simulink model "ss1_inter"  (R2019a)
settings: Solver=ode14x  StartTime=beginTime  StopTime=0.456  FixedStep=1e-4  RelTol=1e-3  EnableMultiTasking=on
model workspace (MAT data in the model file):
  Ankle_L_D = 1.86999822456
  Ankle_L_S = 0.0237763920936
  Ankle_R_D = 0.0588397140494
  Ankle_R_S = 0.739584271752
  F_C = 0.06105
  F_H = 0.07
  F_I = 0.00125071180063
  F_L = 0.185
  F_M = 1.13129
  F_W = 0.1
  GRF_HD = 42097.5090581
  GRF_HS = 111995.804745
  GRF_VD = 23523.4518935
  GRF_VS = 88551.3661398
  HAT_I = 3.41998320224
  HAT_L = 0.51264
  HAT_M = 52.89756
  HAT_a = 0.2
  HAT_b = 0.11
  Hip_L_D = 0.00120944164738
  Hip_L_S = 1.91959156409
  Hip_R_D = 0.00174333284727
  Hip_R_S = 0.483982271561
  Knee_L_D = 0.900041230997
  Knee_L_S = 0.0187606009115
  Knee_R_D = 0.0722123401531
  Knee_R_S = 0.0187606009115
  M : struct (value not decoded)
  S_I = 0.0556212184297
  S_L = 0.41
  S_M = 3.62793
  S_R1 = 0.035
  S_R2 = 0.0716197243914
  T_I = 0.63371745
  T_L = 0.6
  T_M = 7.802
  T_R1 = 0.0716197243914
  T_R2 = 0.105042262441
  beginTime = 0.4399
  bodymass = 78.02
  lagStanceAnkle = [0 0 0 0 0 0]
  lagSwingAnkle = [0 0 0 0 0 0]
  lagSwingHip = [0 0 0 0 0 0]
  lagSwingKnee = [0 0 0 0 0 0]
  p_stance_ankle_i = 17.5320951874
  p_stance_hip_i = 9.45550537668
  p_stance_knee_i = -16.7757020207
  p_swing_ankle_i = -28.2787898978
  p_swing_hip_i = -5.22071177476
  p_swing_knee_i = -39.2892116907
  polyfit_stance_ankle = [7.25005766341 -2.94260084728 3.61751641686 -0.1600680665]
  polyfit_swing_ankle = [-11368.0037517 20285.4827832 -14825.218273 5697.61347658 -1221.0674564 140.988649334 -7.60353693637 0.110238664523]
  polyfit_swing_hip = [-6497.04836191 6353.1189755 -1512.41069047 -218.046365216 114.745718447 -9.14187395017 -0.14056630138]
  polyfit_swing_knee = [20801.7792641 -51031.8985583 53804.8965773 -29864.6420618 9069.83319333 -1458.09150169 107.955966741 -2.65469998779 0.0787369748099]
  w_stance_ankle_i = 0.530344461508
  w_stance_hip_i = -152.886101178
  w_stance_knee_i = 28.9894830902
  w_swing_ankle_i = -177.193414919
  w_swing_hip_i = 0.0149454586906
  w_swing_knee_i = 289.013531197
  x_planar_p_i = -0.0011974861006
  x_planar_v_i = 0.0137263009297
  y_planar_p_i = 0.0112183968788
  y_planar_v_i = -0.080280250047
  z_planar_p_i = 11.2224967124
  z_planar_v_i = -77.4143532804
symbols that are objects in the model workspace (value not decoded): M
undefined symbols (not defined in the file or in its folder): X, Y, Z
libraries: nesl_utility x54, sm_lib x46, fl_lib x24, fl_ps_legacy_lib x14
(part 5 of 7)

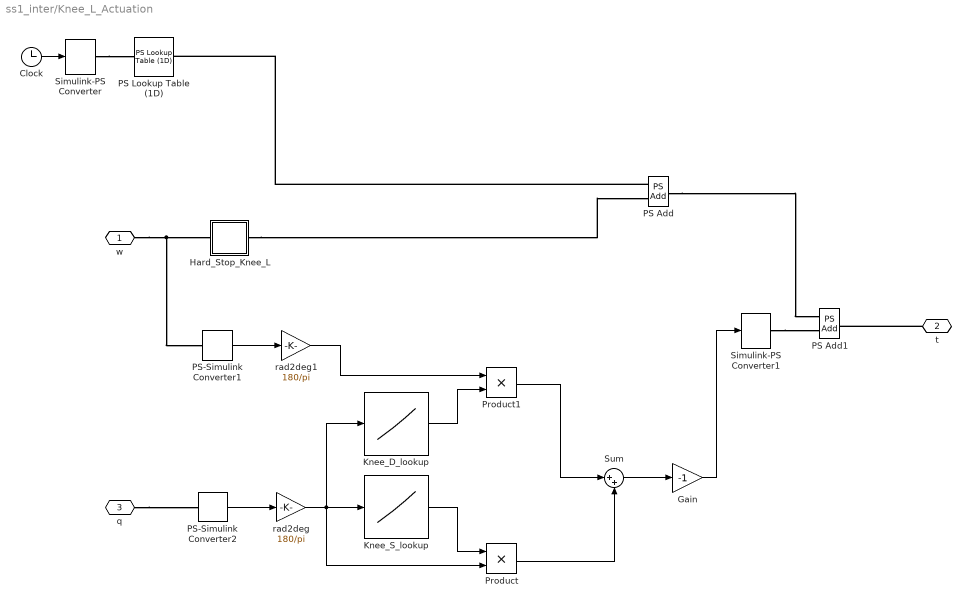
== system ss1_inter/Knee_L_Actuation ==
  Clock : Clock
  Gain : Gain  Gain=-1
  Hard_Stop_Knee_L : Subsystem  mask{upper_bound=(-p_stance_knee_i*pi)/180, lower_bound=((-140-p_stance_knee_i)*pi)/180, contact_stiffness=1e8, contact_damping=5000, initial_angular_position=0}
      mask prompts: upper_bound "Upper Bound"; lower_bound "Lower Bound"; contact_stiffness "Contact Stiffness"; contact_damping "Contact Damping"; initial_angular_position "Initial Angular Position"
  Knee_D_lookup : Lookup_n-D  NumberOfTableDimensions=1  BreakpointsForDimension1=[-140:.01:0]  Table=[exp(linspace(log(1000),log(.01),1000)), zeros(1,12000),exp(linspace(log(.01),log(1000),1001))]  RndMeth=Simplest  InputSameDT=on
  Knee_S_lookup : Lookup_n-D  NumberOfTableDimensions=1  BreakpointsForDimension1=[-140:.01:0]  Table=[exp(linspace(log(10000),log(.01),1000)), zeros(1,12000),exp(linspace(log(.01),log(10000),1001))]  RndMeth=Simplest  InputSameDT=on
  PS Add : fl_ps_legacy_lib/Legacy Physical Signals/Functions/PS Add
      settings: SourceProductName=Simscape  SourceProductBaseCode=SS
  PS Add1 : fl_ps_legacy_lib/Legacy Physical Signals/Functions/PS Add
      settings: SourceProductName=Simscape  SourceProductBaseCode=SS
  PS Lookup Table (1D) : fl_ps_legacy_lib/Legacy Physical Signals/Lookup Tables/PS Lookup Table (1D)  x=linspace(0,.3917,47)'  f=(-M.stance_knee_av/1000)*bodymass  interp_method=2  extrap_method=1
      settings: SourceProductName=Simscape  SourceProductBaseCode=SS
  PS-Simulink Converter1 : nesl_utility/PS-Simulink Converter  PhysicalDomain=network_engine_domain  SubClassName=ps_output  LeftPortType=input  RightPortType=output  PseudoPeriodic=off  Frequencies=[]  Unit=1  AffineConversion=off
  PS-Simulink Converter2 : nesl_utility/PS-Simulink Converter  PhysicalDomain=network_engine_domain  SubClassName=ps_output  LeftPortType=input  RightPortType=output  PseudoPeriodic=off  Frequencies=[]  Unit=1  AffineConversion=off
  Product : Product  RndMeth=Zero
  Product1 : Product  RndMeth=Zero
  Simulink-PS Converter : nesl_utility/Simulink-PS Converter  PhysicalDomain=network_engine_domain  SubClassName=ps_input  LeftPortType=input  RightPortType=output  PseudoPeriodic=off  Frequencies=[]  NoiseDistribution=none  NoiseParameters=[]  Unit=1  AffineConversion=off  FilteringAndDerivatives=zero  SimscapeFilterOrder=1  InputFilterTimeConstant=.001  UdotUserProvided=[]
  Simulink-PS Converter1 : nesl_utility/Simulink-PS Converter  PhysicalDomain=network_engine_domain  SubClassName=ps_input  LeftPortType=input  RightPortType=output  PseudoPeriodic=off  Frequencies=[]  NoiseDistribution=none  NoiseParameters=[]  Unit=1  AffineConversion=off  FilteringAndDerivatives=zero  SimscapeFilterOrder=1  InputFilterTimeConstant=.001  UdotUserProvided=[]
  Sum : Sum  Inputs=|++
  rad2deg : Gain  Gain=180/pi
  "rad2deg1 " : Gain  Gain=180/pi
  w : PMIOPort  Side=Right
  t : PMIOPort  Port=2  Side=Left
  q : PMIOPort  Port=3  Side=Right
  wires:
  Clock/1 -> Simulink-PS Converter/1
  PS-Simulink Converter1/1 -> "rad2deg1 "/1
  PS-Simulink Converter2/1 -> rad2deg/1
  rad2deg/1 -> Knee_S_lookup/1, Knee_D_lookup/1, Product/2
  Knee_S_lookup/1 -> Product/1
  "rad2deg1 "/1 -> Product1/1
  Product1/1 -> Sum/1
  Product/1 -> Sum/2
  Sum/1 -> Gain/1
  Gain/1 -> Simulink-PS Converter1/1
  Knee_D_lookup/1 -> Product1/2
  connections:
  Hard_Stop_Knee_L/RConn1 -- PS Add/LConn2
  w/RConn1 -- PS-Simulink Converter1/LConn1 -- Hard_Stop_Knee_L/LConn1
  Simulink-PS Converter/RConn1 -- PS Lookup Table (1D)/LConn1
  t/RConn1 -- PS Add1/RConn1
  q/RConn1 -- PS-Simulink Converter2/LConn1
  PS Add/RConn1 -- PS Add1/LConn1
  Simulink-PS Converter1/RConn1 -- PS Add1/LConn2
  PS Add/LConn1 -- PS Lookup Table (1D)/RConn1

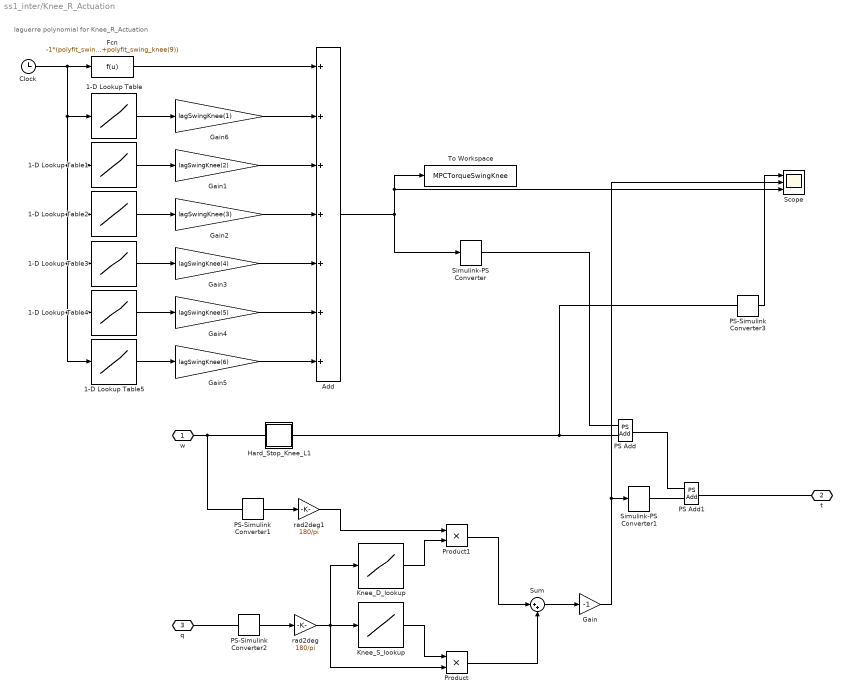
== system ss1_inter/Knee_R_Actuation ==
  note: laguerre polynomial for Knee_R_Actuation
  1-D Lookup Table : Lookup_n-D  NumberOfTableDimensions=1  BreakpointsForDimension1=|  Table=|  InternalRulePriority=Speed  RndMeth=Simplest  InputSameDT=on
      BreakpointsForDimension1=|
      | [0
      | 0.00500000000000000
      | 0.0100000000000000
      | 0.0150000000000000
      | 0.0200000000000000
      | 0.0250000000000000
      | 0.0300000000000000
      | 0.0350000000000000
      | 0.0400000000000000
      | 0.0450000000000000
      | 0.0500000000000000
      | 0.0550000000000000
      | 0.0600000000000000
      | 0.0650000000000000
      | 0.0700000000000000
      | 0.0750000000000000
      | 0.0800000000000000
      | 0.0850000000000000
      | 0.0900000000000000
      | 0.0950000000000000
      | 0.100000000000000
      | 0.105000000000000
      | 0.110000000000000
      | 0.115000000000000
      | 0.120000000000000
      | 0.125000000000000
      | 0.130000000000000
      | 0.135000000000000
      | 0.140000000000000
      | 0.145000000000000
      | 0.150000000000000
      | 0.155000000000000
      | 0.160000000000000
      | 0.165000000000000
      | 0.170000000000000
      | 0.175000000000000
      | 0.180000000000000
      | 0.185000000000000
      | 0.190000000000000
      | 0.195000000000000
      | 0.200000000000000
      | 0.205000000000000
      | 0.210000000000000
      | 0.215000000000000
      | 0.220000000000000
      | 0.225000000000000
      | 0.230000000000000
      | 0.235000000000000
      | 0.240000000000000
      | 0.245000000000000
      | 0.250000000000000
      | 0.255000000000000
      | 0.260000000000000
      | 0.265000000000000
      | 0.270000000000000
      | 0.275000000000000
      | 0.280000000000000
      | 0.285000000000000
      | 0.290000000000000
      | 0.295000000000000
      | 0.300000000000000
      | 0.305000000000000
      | 0.310000000000000
      | 0.315000000000000
      | 0.320000000000000
      | 0.325000000000000
      | 0.330000000000000
      | 0.335000000000000
      | 0.340000000000000
      | 0.345000000000000
      | 0.350000000000000
      | 0.355000000000000
      | 0.360000000000000
      | 0.365000000000000
      | 0.370000000000000
      | 0.375000000000000
      | 0.380000000000000
      | 0.385000000000000
      | 0.390000000000000
      | 0.395000000000000
      | 0.400000000000000
      | 0.405000000000000
      | 0.410000000000000
      | 0.415000000000000
      | 0.420000000000000
      | 0.425000000000000
      | 0.430000000000000
      | 0.435000000000000
      | 0.440000000000000
      | 0.445000000000000
      | 0.450000000000000
      | 0.455000000000000
      | 0.460000000000000
      | 0.465000000000000
      | 0.470000000000000
      | 0.475000000000000
      | 0.480000000000000
      | 0.485000000000000
      | 0.490000000000000
      | 0.495000000000000
      | 0.500000000000000]
      Table=|
      | [0.600000000000000
      | 0.480000000000000
      | 0.384000000000000
      | 0.307200000000000
      | 0.245760000000000
      | 0.196608000000000
      | 0.157286400000000
      | 0.125829120000000
      | 0.100663296000000
      | 0.0805306368000000
      | 0.0644245094400000
      | 0.0515396075520000
      | 0.0412316860416000
      | 0.0329853488332800
      | 0.0263882790666240
      | 0.0211106232532992
      | 0.0168884986026394
      | 0.0135107988821115
      | 0.0108086391056892
      | 0.00864691128455136
      | 0.00691752902764109
      | 0.00553402322211287
      | 0.00442721857769030
      | 0.00354177486215224
      | 0.00283341988972179
      | 0.00226673591177743
      | 0.00181338872942195
      | 0.00145071098353756
      | 0.00116056878683005
      | 0.000928455029464037
      | 0.000742764023571229
      | 0.000594211218856984
      | 0.000475368975085587
      | 0.000380295180068470
      | 0.000304236144054776
      | 0.000243388915243821
      | 0.000194711132195056
      | 0.000155768905756045
      | 0.000124615124604836
      | 9.96920996838689e-05
      | 7.97536797470952e-05
      | 6.38029437976761e-05
      | 5.10423550381409e-05
      | 4.08338840305127e-05
      | 3.26671072244102e-05
      | 2.61336857795281e-05
      | 2.09069486236225e-05
      | 1.67255588988980e-05
      | 1.33804471191184e-05
      | 1.07043576952947e-05
      | 8.56348615623579e-06
      | 6.85078892498863e-06
      | 5.48063113999090e-06
      | 4.38450491199272e-06
      | 3.50760392959418e-06
      | 2.80608314367534e-06
      | 2.24486651494027e-06
      | 1.79589321195222e-06
      | 1.43671456956178e-06
      | 1.14937165564942e-06
      | 9.19497324519537e-07
      | 7.35597859615629e-07
      | 5.88478287692504e-07
      | 4.70782630154003e-07
      | 3.76626104123202e-07
      | 3.01300883298562e-07
      | 2.41040706638850e-07
      | 1.92832565311080e-07
      | 1.54266052248864e-07
      | 1.23412841799091e-07
      | 9.87302734392728e-08
      | 7.89842187514182e-08
      | 6.31873750011346e-08
      | 5.05499000009077e-08
      | 4.04399200007261e-08
      | 3.23519360005809e-08
      | 2.58815488004647e-08
      | 2.07052390403718e-08
      | 1.65641912322974e-08
      | 1.32513529858379e-08
      | 1.06010823886704e-08
      | 8.48086591093629e-09
      | 6.78469272874903e-09
      | 5.42775418299922e-09
      | 4.34220334639938e-09
      | 3.47376267711950e-09
      | 2.77901014169560e-09
      | 2.22320811335648e-09
      | 1.77856649068519e-09
      | 1.42285319254815e-09
      | 1.13828255403852e-09
      | 9.10626043230815e-10
      | 7.28500834584652e-10
      | 5.82800667667722e-10
      | 4.66240534134178e-10
      | 3.72992427307342e-10
      | 2.98393941845874e-10
      | 2.38715153476699e-10
      | 1.90972122781359e-10
      | 1.52777698225087e-10
      | 1.22222158580070e-10]
  1-D Lookup Table1 : Lookup_n-D  NumberOfTableDimensions=1  BreakpointsForDimension1=|  Table=|  InternalRulePriority=Speed  RndMeth=Simplest  InputSameDT=on
      BreakpointsForDimension1=|
      | [0
      | 0.00500000000000000
      | 0.0100000000000000
      | 0.0150000000000000
      | 0.0200000000000000
      | 0.0250000000000000
      | 0.0300000000000000
      | 0.0350000000000000
      | 0.0400000000000000
      | 0.0450000000000000
      | 0.0500000000000000
      | 0.0550000000000000
      | 0.0600000000000000
      | 0.0650000000000000
      | 0.0700000000000000
      | 0.0750000000000000
      | 0.0800000000000000
      | 0.0850000000000000
      | 0.0900000000000000
      | 0.0950000000000000
      | 0.100000000000000
      | 0.105000000000000
      | 0.110000000000000
      | 0.115000000000000
      | 0.120000000000000
      | 0.125000000000000
      | 0.130000000000000
      | 0.135000000000000
      | 0.140000000000000
      | 0.145000000000000
      | 0.150000000000000
      | 0.155000000000000
      | 0.160000000000000
      | 0.165000000000000
      | 0.170000000000000
      | 0.175000000000000
      | 0.180000000000000
      | 0.185000000000000
      | 0.190000000000000
      | 0.195000000000000
      | 0.200000000000000
      | 0.205000000000000
      | 0.210000000000000
      | 0.215000000000000
      | 0.220000000000000
      | 0.225000000000000
      | 0.230000000000000
      | 0.235000000000000
      | 0.240000000000000
      | 0.245000000000000
      | 0.250000000000000
      | 0.255000000000000
      | 0.260000000000000
      | 0.265000000000000
      | 0.270000000000000
      | 0.275000000000000
      | 0.280000000000000
      | 0.285000000000000
      | 0.290000000000000
      | 0.295000000000000
      | 0.300000000000000
      | 0.305000000000000
      | 0.310000000000000
      | 0.315000000000000
      | 0.320000000000000
      | 0.325000000000000
      | 0.330000000000000
      | 0.335000000000000
      | 0.340000000000000
      | 0.345000000000000
      | 0.350000000000000
      | 0.355000000000000
      | 0.360000000000000
      | 0.365000000000000
      | 0.370000000000000
      | 0.375000000000000
      | 0.380000000000000
      | 0.385000000000000
      | 0.390000000000000
      | 0.395000000000000
      | 0.400000000000000
      | 0.405000000000000
      | 0.410000000000000
      | 0.415000000000000
      | 0.420000000000000
      | 0.425000000000000
      | 0.430000000000000
      | 0.435000000000000
      | 0.440000000000000
      | 0.445000000000000
      | 0.450000000000000
      | 0.455000000000000
      | 0.460000000000000
      | 0.465000000000000
      | 0.470000000000000
      | 0.475000000000000
      | 0.480000000000000
      | 0.485000000000000
      | 0.490000000000000
      | 0.495000000000000
      | 0.500000000000000]
      Table=|
      | [-0.480000000000000
      | -0.168000000000000
      | 0.0383999999999999
      | 0.168960000000000
      | 0.245760000000000
      | 0.285081600000000
      | 0.298844160000000
      | 0.295698432000000
      | 0.281857228800000
      | 0.261724569600000
      | 0.238370684928000
      | 0.213889371340800
      | 0.189665755791360
      | 0.166576011608064
      | 0.145135534866432
      | 0.125608208357130
      | 0.108086391056892
      | 0.0925489723424637
      | 0.0789030654715311
      | 0.0670135624552730
      | 0.0567237380266569
      | 0.0478693008712763
      | 0.0402876890569817
      | 0.0338239499335539
      | 0.0283341988972179
      | 0.0236873902780742
      | 0.0197659371506992
      | 0.0164655696631513
      | 0.0136947116845945
      | 0.0113735741109344
      | 0.00943310309935461
      | 0.00781387752796933
      | 0.00646501806116398
      | 0.00534314727996199
      | 0.00441142408879424
      | 0.00363866428289511
      | 0.00299855143580387
      | 0.00246893715623331
      | 0.00203122653105883
      | 0.00166984266970480
      | 0.00137176329165004
      | 0.00112612195802898
      | 0.000923866626190350
      | 0.000757468548766011
      | 0.000620675037263793
      | 0.000508300188411822
      | 0.000416048277610088
      | 0.000340365123592574
      | 0.000278313300077663
      | 0.000227467601025013
      | 0.000185827649590316
      | 0.000151744974688498
      | 0.000123862263763794
      | 0.000101062838221432
      | 8.24286923454631e-05
      | 6.72056912910244e-05
      | 5.47747429645427e-05
      | 4.46279463170126e-05
      | 3.63488786099129e-05
      | 2.95963201329726e-05
      | 2.40908299024118e-05
      | 1.96036829587565e-05
      | 1.59477615964668e-05
      | 1.29700614607428e-05
      | 1.05455309154497e-05
      | 8.57201012984408e-06
      | 6.96607642186275e-06
      | 5.65963579188018e-06
      | 4.59712835701614e-06
      | 3.73323846442250e-06
      | 3.03101939458567e-06
      | 2.46035841410668e-06
      | 1.99672105003585e-06
      | 1.62012429502909e-06
      | 1.31429740002360e-06
      | 1.06599629121914e-06
      | 8.64443729935521e-07
      | 7.00872341516584e-07
      | 5.68151759267801e-07
      | 4.60484516257868e-07
      | 3.73158100081196e-07
      | 3.02342869724878e-07
      | 2.44927407507840e-07
      | 1.98384415388621e-07
      | 1.60661523816777e-07
      | 1.30092412258125e-07
      | 1.05324484370263e-07
      | 8.52600311472210e-08
      | 6.90083798385852e-08
      | 5.58469878075148e-08
      | 4.51898173953292e-08
      | 3.65616356357172e-08
      | 2.95771338841369e-08
      | 2.39239674077600e-08
      | 1.93489821665684e-08
      | 1.56470323255430e-08
      | 1.26519031342650e-08
      | 1.02289443264765e-08
      | 8.26909291643285e-09
      | 6.68402429734757e-09
      | 5.40221940923909e-09]
  1-D Lookup Table2 : Lookup_n-D  NumberOfTableDimensions=1  BreakpointsForDimension1=|  Table=|  InternalRulePriority=Speed  RndMeth=Simplest  InputSameDT=on
      BreakpointsForDimension1=|
      | [0
      | 0.00500000000000000
      | 0.0100000000000000
      | 0.0150000000000000
      | 0.0200000000000000
      | 0.0250000000000000
      | 0.0300000000000000
      | 0.0350000000000000
      | 0.0400000000000000
      | 0.0450000000000000
      | 0.0500000000000000
      | 0.0550000000000000
      | 0.0600000000000000
      | 0.0650000000000000
      | 0.0700000000000000
      | 0.0750000000000000
      | 0.0800000000000000
      | 0.0850000000000000
      | 0.0900000000000000
      | 0.0950000000000000
      | 0.100000000000000
      | 0.105000000000000
      | 0.110000000000000
      | 0.115000000000000
      | 0.120000000000000
      | 0.125000000000000
      | 0.130000000000000
      | 0.135000000000000
      | 0.140000000000000
      | 0.145000000000000
      | 0.150000000000000
      | 0.155000000000000
      | 0.160000000000000
      | 0.165000000000000
      | 0.170000000000000
      | 0.175000000000000
      | 0.180000000000000
      | 0.185000000000000
      | 0.190000000000000
      | 0.195000000000000
      | 0.200000000000000
      | 0.205000000000000
      | 0.210000000000000
      | 0.215000000000000
      | 0.220000000000000
      | 0.225000000000000
      | 0.230000000000000
      | 0.235000000000000
      | 0.240000000000000
      | 0.245000000000000
      | 0.250000000000000
      | 0.255000000000000
      | 0.260000000000000
      | 0.265000000000000
      | 0.270000000000000
      | 0.275000000000000
      | 0.280000000000000
      | 0.285000000000000
      | 0.290000000000000
      | 0.295000000000000
      | 0.300000000000000
      | 0.305000000000000
      | 0.310000000000000
      | 0.315000000000000
      | 0.320000000000000
      | 0.325000000000000
      | 0.330000000000000
      | 0.335000000000000
      | 0.340000000000000
      | 0.345000000000000
      | 0.350000000000000
      | 0.355000000000000
      | 0.360000000000000
      | 0.365000000000000
      | 0.370000000000000
      | 0.375000000000000
      | 0.380000000000000
      | 0.385000000000000
      | 0.390000000000000
      | 0.395000000000000
      | 0.400000000000000
      | 0.405000000000000
      | 0.410000000000000
      | 0.415000000000000
      | 0.420000000000000
      | 0.425000000000000
      | 0.430000000000000
      | 0.435000000000000
      | 0.440000000000000
      | 0.445000000000000
      | 0.450000000000000
      | 0.455000000000000
      | 0.460000000000000
      | 0.465000000000000
      | 0.470000000000000
      | 0.475000000000000
      | 0.480000000000000
      | 0.485000000000000
      | 0.490000000000000
      | 0.495000000000000
      | 0.500000000000000]
      Table=|
      | [0.384000000000000
      | -0.0383999999999998
      | -0.229440000000000
      | -0.280320000000000
      | -0.251904000000000
      | -0.183828480000000
      | -0.101056512000000
      | -0.0185597952000002
      | 0.0553648127999998
      | 0.116769423360000
      | 0.164443560345600
      | 0.198814036131840
      | 0.221207995613184
      | 0.233371342995456
      | 0.237164658111283
      | 0.234380694669754
      | 0.226643651247420
      | 0.215362134180857
      | 0.201716227309924
      | 0.186665197355252
      | 0.170966729918149
      | 0.155201681264155
      | 0.139800494637015
      | 0.125068924819751
      | 0.111211730671580
      | 0.0983536712120227
      | 0.0865575775271329
      | 0.0758395434418845
      | 0.0661814350689833
      | 0.0575410004510336
      | 0.0498598919922776
      | 0.0430699146708013
      | 0.0370977948156792
      | 0.0318687360897377
      | 0.0273089968807168
      | 0.0233476901670516
      | 0.0199179752678933
      | 0.0169577819251318
      | 0.0144101814714917
      | 0.0122234975724884
      | 0.0103512300943755
      | 0.00875184980072722
      | 0.00738850849765848
      | 0.00622869858530433
      | 0.00524388738719844
      | 0.00440914479629309
      | 0.00370277740335822
      | 0.00310597810142260
      | 0.00260249696466853
      | 0.00217833679099247
      | 0.00182147491414674
      | 0.00152161160115691
      | 0.00126994444460299
      | 0.00105896754886904
      | 0.000882293923440294
      | 0.000734499278064879
      | 0.000610985319371294
      | 0.000507860641407968
      | 0.000421837356555456
      | 0.000350141707747900
      | 0.000290437022409363
      | 0.000240757501462897
      | 0.000199451474851901
      | 0.000165132892309393
      | 0.000136639950575898
      | 0.000112999883272293
      | 9.33990556101879e-05
      | 7.71576122765089e-05
      | 6.37080229274744e-05
      | 5.25769559274577e-05
      | 4.33699876907201e-05
      | 3.57587228158764e-05
      | 2.94699598267791e-05
      | 2.42765894754359e-05
      | 1.99899579553589e-05
      | 1.64534667313354e-05
      | 1.35372146923391e-05
      | 1.11335176105935e-05
      | 9.15316502257715e-06
      | 7.52229616432322e-06
      | 6.17979496765149e-06
      | 5.07511977842249e-06
      | 4.16649676645660e-06
      | 3.41941728836222e-06
      | 2.80538902702498e-06
      | 2.30089881563026e-06
      | 1.88655187726612e-06
      | 1.54635796126538e-06
      | 1.26713969628866e-06
      | 1.03804254662350e-06
      | 8.50129171190052e-07
      | 6.96043845838798e-07
      | 5.69735005199446e-07
      | 4.66225964117485e-07
      | 3.81425552968494e-07
      | 3.11971798680929e-07
      | 2.55102948762874e-07
      | 2.08551106683383e-07
      | 1.70454555340037e-07
      | 1.39285517750584e-07
      | 1.13790662970424e-07]
  1-D Lookup Table3 : Lookup_n-D  NumberOfTableDimensions=1  BreakpointsForDimension1=|  Table=|  InternalRulePriority=Speed  RndMeth=Simplest  InputSameDT=on
      BreakpointsForDimension1=|
      | [0
      | 0.00500000000000000
      | 0.0100000000000000
      | 0.0150000000000000
      | 0.0200000000000000
      | 0.0250000000000000
      | 0.0300000000000000
      | 0.0350000000000000
      | 0.0400000000000000
      | 0.0450000000000000
      | 0.0500000000000000
      | 0.0550000000000000
      | 0.0600000000000000
      | 0.0650000000000000
      | 0.0700000000000000
      | 0.0750000000000000
      | 0.0800000000000000
      | 0.0850000000000000
      | 0.0900000000000000
      | 0.0950000000000000
      | 0.100000000000000
      | 0.105000000000000
      | 0.110000000000000
      | 0.115000000000000
      | 0.120000000000000
      | 0.125000000000000
      | 0.130000000000000
      | 0.135000000000000
      | 0.140000000000000
      | 0.145000000000000
      | 0.150000000000000
      | 0.155000000000000
      | 0.160000000000000
      | 0.165000000000000
      | 0.170000000000000
      | 0.175000000000000
      | 0.180000000000000
      | 0.185000000000000
      | 0.190000000000000
      | 0.195000000000000
      | 0.200000000000000
      | 0.205000000000000
      | 0.210000000000000
      | 0.215000000000000
      | 0.220000000000000
      | 0.225000000000000
      | 0.230000000000000
      | 0.235000000000000
      | 0.240000000000000
      | 0.245000000000000
      | 0.250000000000000
      | 0.255000000000000
      | 0.260000000000000
      | 0.265000000000000
      | 0.270000000000000
      | 0.275000000000000
      | 0.280000000000000
      | 0.285000000000000
      | 0.290000000000000
      | 0.295000000000000
      | 0.300000000000000
      | 0.305000000000000
      | 0.310000000000000
      | 0.315000000000000
      | 0.320000000000000
      | 0.325000000000000
      | 0.330000000000000
      | 0.335000000000000
      | 0.340000000000000
      | 0.345000000000000
      | 0.350000000000000
      | 0.355000000000000
      | 0.360000000000000
      | 0.365000000000000
      | 0.370000000000000
      | 0.375000000000000
      | 0.380000000000000
      | 0.385000000000000
      | 0.390000000000000
      | 0.395000000000000
      | 0.400000000000000
      | 0.405000000000000
      | 0.410000000000000
      | 0.415000000000000
      | 0.420000000000000
      | 0.425000000000000
      | 0.430000000000000
      | 0.435000000000000
      | 0.440000000000000
      | 0.445000000000000
      | 0.450000000000000
      | 0.455000000000000
      | 0.460000000000000
      | 0.465000000000000
      | 0.470000000000000
      | 0.475000000000000
      | 0.480000000000000
      | 0.485000000000000
      | 0.490000000000000
      | 0.495000000000000
      | 0.500000000000000]
      Table=|
      | [-0.307200000000000
      | 0.168960000000000
      | 0.280320000000000
      | 0.219072000000000
      | 0.0964608000000002
      | -0.0276725759999998
      | -0.125121331200000
      | -0.186305740800000
      | -0.211896238080000
      | -0.207567716352000
      | -0.180839597998080
      | -0.139279346958336
      | -0.0895758379253762
      | -0.0371497491234818
      | 0.0139198172076439
      | 0.0607959561415948
      | 0.101702538585094
      | 0.135715974770810
      | 0.162561932149565
      | 0.182433615145375
      | 0.195838705537033
      | 0.203476349336451
      | 0.206142365023704
      | 0.204659246800178
      | 0.199826937722629
      | 0.192390343880065
      | 0.183019884294368
      | 0.172301850209120
      | 0.160735875553994
      | 0.148737335151352
      | 0.136642954978293
      | 0.124718324238271
      | 0.113166338208875
      | 0.102135876510989
      | 0.0917302397939552
      | 0.0820150365822397
      | 0.0730253392185287
      | 0.0647720211026108
      | 0.0572472536300271
      | 0.0504291863175227
      | 0.0442858625510061
      | 0.0387784402945986
      | 0.0338637952382793
      | 0.0294965858200385
      | 0.0256308573315764
      | 0.0222212574154251
      | 0.0192239288059466
      | 0.0165971379669774
      | 0.0143016909032697
      | 0.0123011802544903
      | 0.0105621010632673
      | 0.00905386648383507
      | 0.00774874923254257
      | 0.00662176979154182
      | 0.00565054824335026
      | 0.00481513309566860
      | 0.00409781749910272
      | 0.00348295080552710
      | 0.00295675140058528
      | 0.00250712511082536
      | 0.00212349217848070
      | 0.00179662476402360
      | 0.00151849613280026
      | 0.00128214206724459
      | 0.00108153458564435
      | 0.000911467712473544
      | 0.000767454808762978
      | 0.000645636812799363
      | 0.000542700644174020
      | 0.000455806973524724
      | 0.000382526544594661
      | 0.000320784245113748
      | 0.000268810151045451
      | 0.000225096809082792
      | 0.000188362070377382
      | 0.000157516840872196
      | 0.000131637167675221
      | 0.000109940134744041
      | 9.17630933877647e-05
      | 7.65458028013303e-05
      | 6.38151024312663e-05
      | 5.31717810899266e-05
      | 4.42793472371985e-05
      | 3.68544407255256e-05
      | 3.06586586471627e-05
      | 2.54915968922509e-05
      | 2.11849348276181e-05
      | 1.75974133703483e-05
      | 1.46105769005131e-05
      | 1.21251671794003e-05
      | 1.00580729531917e-05
      | 8.33975245707240e-06
      | 6.91205780733716e-06
      | 5.72640047977519e-06
      | 4.74220590556284e-06
      | 3.92561283847402e-06
      | 3.24837971044985e-06
      | 2.68696583177605e-06
      | 2.22176012783219e-06
      | 1.83643424340532e-06
      | 1.51740038209850e-06]
  1-D Lookup Table4 : Lookup_n-D  NumberOfTableDimensions=1  BreakpointsForDimension1=|  Table=|  InternalRulePriority=Speed  RndMeth=Simplest  InputSameDT=on
      BreakpointsForDimension1=|
      | [0
      | 0.00500000000000000
      | 0.0100000000000000
      | 0.0150000000000000
      | 0.0200000000000000
      | 0.0250000000000000
      | 0.0300000000000000
      | 0.0350000000000000
      | 0.0400000000000000
      | 0.0450000000000000
      | 0.0500000000000000
      | 0.0550000000000000
      | 0.0600000000000000
      | 0.0650000000000000
      | 0.0700000000000000
      | 0.0750000000000000
      | 0.0800000000000000
      | 0.0850000000000000
      | 0.0900000000000000
      | 0.0950000000000000
      | 0.100000000000000
      | 0.105000000000000
      | 0.110000000000000
      | 0.115000000000000
      | 0.120000000000000
      | 0.125000000000000
      | 0.130000000000000
      | 0.135000000000000
      | 0.140000000000000
      | 0.145000000000000
      | 0.150000000000000
      | 0.155000000000000
      | 0.160000000000000
      | 0.165000000000000
      | 0.170000000000000
      | 0.175000000000000
      | 0.180000000000000
      | 0.185000000000000
      | 0.190000000000000
      | 0.195000000000000
      | 0.200000000000000
      | 0.205000000000000
      | 0.210000000000000
      | 0.215000000000000
      | 0.220000000000000
      | 0.225000000000000
      | 0.230000000000000
      | 0.235000000000000
      | 0.240000000000000
      | 0.245000000000000
      | 0.250000000000000
      | 0.255000000000000
      | 0.260000000000000
      | 0.265000000000000
      | 0.270000000000000
      | 0.275000000000000
      | 0.280000000000000
      | 0.285000000000000
      | 0.290000000000000
      | 0.295000000000000
      | 0.300000000000000
      | 0.305000000000000
      | 0.310000000000000
      | 0.315000000000000
      | 0.320000000000000
      | 0.325000000000000
      | 0.330000000000000
      | 0.335000000000000
      | 0.340000000000000
      | 0.345000000000000
      | 0.350000000000000
      | 0.355000000000000
      | 0.360000000000000
      | 0.365000000000000
      | 0.370000000000000
      | 0.375000000000000
      | 0.380000000000000
      | 0.385000000000000
      | 0.390000000000000
      | 0.395000000000000
      | 0.400000000000000
      | 0.405000000000000
      | 0.410000000000000
      | 0.415000000000000
      | 0.420000000000000
      | 0.425000000000000
      | 0.430000000000000
      | 0.435000000000000
      | 0.440000000000000
      | 0.445000000000000
      | 0.450000000000000
      | 0.455000000000000
      | 0.460000000000000
      | 0.465000000000000
      | 0.470000000000000
      | 0.475000000000000
      | 0.480000000000000
      | 0.485000000000000
      | 0.490000000000000
      | 0.495000000000000
      | 0.500000000000000]
      Table=|
      | [0.245760000000000
      | -0.245760000000000
      | -0.251904000000000
      | -0.0964608000000002
      | 0.0647347199999998
      | 0.170386636800000
      | 0.208733798400000
      | 0.190910300160000
      | 0.135939489792000
      | 0.0629095268352003
      | -0.0125684164853756
      | -0.0794708536197116
      | -0.131195359513804
      | -0.164812326237634
      | -0.180135463879704
      | -0.178825318809395
      | -0.163626329773997
      | -0.137771305050751
      | -0.104550614989443
      | -0.0670254519582894
      | -0.0278577108508829
      | 0.0107714573871654
      | 0.0471796232272202
      | 0.0801586661653380
      | 0.108924629554345
      | 0.133054366262053
      | 0.152417929454213
      | 0.167112747690443
      | 0.177403347918279
      | 0.183668685767536
      | 0.186357919782746
      | 0.185954631413873
      | 0.182948958802269
      | 0.177816804041899
      | 0.171005127909344
      | 0.162922312855639
      | 0.153932615491928
      | 0.144353814729982
      | 0.134457269982575
      | 0.124469720562069
      | 0.114576272726373
      | 0.104924128496425
      | 0.0956267069011156
      | 0.0867678921031410
      | 0.0784062136372902
      | 0.0705788223090684
      | 0.0633051722179226
      | 0.0565903562067027
      | 0.0504280702097238
      | 0.0448032028674565
      | 0.0396940616978416
      | 0.0350742572344726
      | 0.0309142728853791
      | 0.0271827517076124
      | 0.0238475325629515
      | 0.0208764678171766
      | 0.0182380533501277
      | 0.0159018995347832
      | 0.0138390693128854
      | 0.0120223067622333
      | 0.0104261767778275
      | 0.00902713378952380
      | 0.00780353488940243
      | 0.00673561039052653
      | 0.00580540271115034
      | 0.00499668258458579
      | 0.00429484993313179
      | 0.00368682530502892
      | 0.00316093654148328
      | 0.00270680429854087
      | 0.00231522917668169
      | 0.00197808248984902
      | 0.00168820211615660
      | 0.00143929439670450
      | 0.00122584267014448
      | 0.00104302273379521
      | 0.000886625293768189
      | 0.000752985294894539
      | 0.000638917895949461
      | 0.000541660767906269
      | 0.000458822335181333
      | 0.000388335545704391
      | 0.000328416739863681
      | 0.000277529186547723
      | 0.000234350863045973
      | 0.000197746071570141
      | 0.000166740506286269
      | 0.000140499409160355
      | 0.000118308479178222
      | 9.95572264995701e-05
      | 8.37244900165031e-05
      | 7.03658630007363e-05
      | 5.91027966117917e-05
      | 4.96131747129504e-05
      | 4.16231755256852e-05
      | 3.49002560553318e-05
      | 2.92471139143796e-05
      | 2.44964981765327e-05
      | 2.05067562707364e-05
      | 1.71580177496971e-05
      | 1.43489281374842e-05]
  1-D Lookup Table5 : Lookup_n-D  NumberOfTableDimensions=1  BreakpointsForDimension1=|  Table=|  InternalRulePriority=Speed  RndMeth=Simplest  InputSameDT=on
      BreakpointsForDimension1=|
      | [0
      | 0.00500000000000000
      | 0.0100000000000000
      | 0.0150000000000000
      | 0.0200000000000000
      | 0.0250000000000000
      | 0.0300000000000000
      | 0.0350000000000000
      | 0.0400000000000000
      | 0.0450000000000000
      | 0.0500000000000000
      | 0.0550000000000000
      | 0.0600000000000000
      | 0.0650000000000000
      | 0.0700000000000000
      | 0.0750000000000000
      | 0.0800000000000000
      | 0.0850000000000000
      | 0.0900000000000000
      | 0.0950000000000000
      | 0.100000000000000
      | 0.105000000000000
      | 0.110000000000000
      | 0.115000000000000
      | 0.120000000000000
      | 0.125000000000000
      | 0.130000000000000
      | 0.135000000000000
      | 0.140000000000000
      | 0.145000000000000
      | 0.150000000000000
      | 0.155000000000000
      | 0.160000000000000
      | 0.165000000000000
      | 0.170000000000000
      | 0.175000000000000
      | 0.180000000000000
      | 0.185000000000000
      | 0.190000000000000
      | 0.195000000000000
      | 0.200000000000000
      | 0.205000000000000
      | 0.210000000000000
      | 0.215000000000000
      | 0.220000000000000
      | 0.225000000000000
      | 0.230000000000000
      | 0.235000000000000
      | 0.240000000000000
      | 0.245000000000000
      | 0.250000000000000
      | 0.255000000000000
      | 0.260000000000000
      | 0.265000000000000
      | 0.270000000000000
      | 0.275000000000000
      | 0.280000000000000
      | 0.285000000000000
      | 0.290000000000000
      | 0.295000000000000
      | 0.300000000000000
      | 0.305000000000000
      | 0.310000000000000
      | 0.315000000000000
      | 0.320000000000000
      | 0.325000000000000
      | 0.330000000000000
      | 0.335000000000000
      | 0.340000000000000
      | 0.345000000000000
      | 0.350000000000000
      | 0.355000000000000
      | 0.360000000000000
      | 0.365000000000000
      | 0.370000000000000
      | 0.375000000000000
      | 0.380000000000000
      | 0.385000000000000
      | 0.390000000000000
      | 0.395000000000000
      | 0.400000000000000
      | 0.405000000000000
      | 0.410000000000000
      | 0.415000000000000
      | 0.420000000000000
      | 0.425000000000000
      | 0.430000000000000
      | 0.435000000000000
      | 0.440000000000000
      | 0.445000000000000
      | 0.450000000000000
      | 0.455000000000000
      | 0.460000000000000
      | 0.465000000000000
      | 0.470000000000000
      | 0.475000000000000
      | 0.480000000000000
      | 0.485000000000000
      | 0.490000000000000
      | 0.495000000000000
      | 0.500000000000000]
      Table=|
      | [-0.196608000000000
      | 0.285081600000000
      | 0.183828480000000
      | -0.0276725759999998
      | -0.170386636800000
      | -0.207883898880000
      | -0.162907521024000
      | -0.0743204585472002
      | 0.0227023414886397
      | 0.103773741514752
      | 0.155983253235302
      | 0.175794868998635
      | 0.166121329190240
      | 0.133551564828495
      | 0.0861372967289254
      | 0.0318346285509523
      | -0.0224565521494362
      | -0.0713745274529447
      | -0.111230435021552
      | -0.139914601440054
      | -0.156670964429626
      | -0.161811648304316
      | -0.156421559838064
      | -0.142084557575501
      | -0.120648683538539
      | -0.0940378102861284
      | -0.0641102255302200
      | -0.0325604491223173
      | -0.000858289942034466
      | 0.0297817673506227
      | 0.0584077638218371
      | 0.0843204257091174
      | 0.107051804939351
      | 0.126336959520231
      | 0.142082269330609
      | 0.154333093089320
      | 0.163242694933553
      | 0.169043719654784
      | 0.172022974467749
      | 0.172499873107119
      | 0.170808600866666
      | 0.167283850622565
      | 0.162249843473585
      | 0.156012267997471
      | 0.148852735591286
      | 0.141025344263064
      | 0.132754959945181
      | 0.124236855208706
      | 0.115637384205888
      | 0.107095415280469
      | 0.0987242857335585
      | 0.0906140844971104
      | 0.0828341065238576
      | 0.0754353567383752
      | 0.0684530110479514
      | 0.0619087671475713
      | 0.0558130388551315
      | 0.0501669648064063
      | 0.0449642159295999
      | 0.0401925966467787
      | 0.0358354426573943
      | 0.0318728238721239
      | 0.0282825649757010
      | 0.0250410985575420
      | 0.0221241670676399
      | 0.0195073902975936
      | 0.0171667148761552
      | 0.0150787615900328
      | 0.0132210853438686
      | 0.0115723613777454
      | 0.0101125100593919
      | 0.00882277123231597
      | 0.00768573778277652
      | 0.00668535682501421
      | 0.00580690572060028
      | 0.00503694905958854
      | 0.00436328174645149
      | 0.00377486245501375
      | 0.00326174094214597
      | 0.00281498203534122
      | 0.00242658852803418
      | 0.00208942472104516
      | 0.00179714193064958
      | 0.00154410693514517
      | 0.00132533404422708
      | 0.00113642124117152
      | 0.000973490659478343
      | 0.000833133506540660
      | 0.000712359431050305
      | 0.000608550242818810
      | 0.000519417828741416
      | 0.000442966062609046
      | 0.000377456475798540
      | 0.000321377437480263
      | 0.000273416584276613
      | 0.000232436238102710
      | 0.000197451555405996
      | 0.000167611159697951
      | 0.000142180020918304
      | 0.000120524358805622
      | 0.000102098362284207]
  Add : Sum  Inputs=+++++++
  Clock : Clock
  Fcn : Fcn  Expr=-1*(polyfit_swing_knee(1)*u^8+polyfit_swing_knee(2)*u^7+polyfit_swing_knee(3)*u^6+polyfit_swing_knee(4)*u^5+polyfit_swing_knee(5)*u^4+polyfit_swing_knee(6)*u^3+polyfit_swing_knee(7)*u^2+polyfit_swing_knee(8)*u+polyfit_swing_knee(9))
  Gain : Gain  Gain=-1
  Gain1 : Gain  Gain=lagSwingKnee(2)
  Gain2 : Gain  Gain=lagSwingKnee(3)
  Gain3 : Gain  Gain=lagSwingKnee(4)
  Gain4 : Gain  Gain=lagSwingKnee(5)
  Gain5 : Gain  Gain=lagSwingKnee(6)
  Gain6 : Gain  Gain=lagSwingKnee(1)
  Hard_Stop_Knee_L1 : Subsystem  mask{upper_bound=(-p_swing_knee_i*pi)/180, lower_bound=((-140-p_swing_knee_i)*pi)/180, contact_stiffness=1e8, contact_damping=5000, initial_angular_position=0}
      mask prompts: upper_bound "Upper Bound"; lower_bound "Lower Bound"; contact_stiffness "Contact Stiffness"; contact_damping "Contact Damping"; initial_angular_position "Initial Angular Position"
  Knee_D_lookup : Lookup_n-D  NumberOfTableDimensions=1  BreakpointsForDimension1=[-140:.01:0]  Table=[exp(linspace(log(1000),log(.01),1000)), zeros(1,12000),exp(linspace(log(.01),log(1000),1001))]  RndMeth=Simplest  InputSameDT=on
  Knee_S_lookup : Lookup_n-D  NumberOfTableDimensions=1  BreakpointsForDimension1=[-140:.01:0]  Table=[exp(linspace(log(10000),log(.01),1000)), zeros(1,12000),exp(linspace(log(.01),log(10000),1001))]  RndMeth=Simplest  InputSameDT=on
  PS Add : fl_ps_legacy_lib/Legacy Physical Signals/Functions/PS Add
      settings: SourceProductName=Simscape  SourceProductBaseCode=SS
  PS Add1 : fl_ps_legacy_lib/Legacy Physical Signals/Functions/PS Add
      settings: SourceProductName=Simscape  SourceProductBaseCode=SS
  PS-Simulink Converter1 : nesl_utility/PS-Simulink Converter  PhysicalDomain=network_engine_domain  SubClassName=ps_output  LeftPortType=input  RightPortType=output  PseudoPeriodic=off  Frequencies=[]  Unit=1  AffineConversion=off
  PS-Simulink Converter2 : nesl_utility/PS-Simulink Converter  PhysicalDomain=network_engine_domain  SubClassName=ps_output  LeftPortType=input  RightPortType=output  PseudoPeriodic=off  Frequencies=[]  Unit=1  AffineConversion=off
  PS-Simulink Converter3 : nesl_utility/PS-Simulink Converter  PhysicalDomain=network_engine_domain  SubClassName=ps_output  LeftPortType=input  RightPortType=output  PseudoPeriodic=off  Frequencies=[]  Unit=1  AffineConversion=off
  Product : Product  RndMeth=Zero
  Product1 : Product  RndMeth=Zero
  Scope : Scope  NumInputPorts=3
  Simulink-PS Converter : nesl_utility/Simulink-PS Converter  PhysicalDomain=network_engine_domain  SubClassName=ps_input  LeftPortType=input  RightPortType=output  PseudoPeriodic=off  Frequencies=[]  NoiseDistribution=none  NoiseParameters=[]  Unit=1  AffineConversion=off  FilteringAndDerivatives=zero  SimscapeFilterOrder=1  InputFilterTimeConstant=.001  UdotUserProvided=[]
  Simulink-PS Converter1 : nesl_utility/Simulink-PS Converter  PhysicalDomain=network_engine_domain  SubClassName=ps_input  LeftPortType=input  RightPortType=output  PseudoPeriodic=off  Frequencies=[]  NoiseDistribution=none  NoiseParameters=[]  Unit=1  AffineConversion=off  FilteringAndDerivatives=zero  SimscapeFilterOrder=1  InputFilterTimeConstant=.001  UdotUserProvided=[]
  Sum : Sum  Inputs=|++
  To Workspace : ToWorkspace  VariableName=MPCTorqueSwingKnee  SampleTime=-1
  rad2deg : Gain  Gain=180/pi
  "rad2deg1 " : Gain  Gain=180/pi
  w : PMIOPort  Side=Right
  t : PMIOPort  Port=2  Side=Left
  q : PMIOPort  Port=3  Side=Right
  wires:
  PS-Simulink Converter1/1 -> "rad2deg1 "/1
  PS-Simulink Converter2/1 -> rad2deg/1
  rad2deg/1 -> Knee_D_lookup/1, Knee_S_lookup/1, Product/2
  Knee_S_lookup/1 -> Product/1
  "rad2deg1 "/1 -> Product1/1
  Product1/1 -> Sum/1
  Product/1 -> Sum/2
  Sum/1 -> Gain/1
  Knee_D_lookup/1 -> Product1/2
  Gain5/1 -> Add/7
  1-D Lookup Table5/1 -> Gain5/1
  Gain4/1 -> Add/6
  1-D Lookup Table4/1 -> Gain4/1
  Gain3/1 -> Add/5
  1-D Lookup Table3/1 -> Gain3/1
  Gain2/1 -> Add/4
  1-D Lookup Table2/1 -> Gain2/1
  Gain1/1 -> Add/3
  1-D Lookup Table1/1 -> Gain1/1
  Gain6/1 -> Add/2
  1-D Lookup Table/1 -> Gain6/1
  Clock/1 -> 1-D Lookup Table/1, 1-D Lookup Table1/1, 1-D Lookup Table2/1, 1-D Lookup Table3/1, 1-D Lookup Table5/1, 1-D Lookup Table4/1, Fcn/1
  Gain/1 -> Scope/2, Simulink-PS Converter1/1
  PS-Simulink Converter3/1 -> Scope/1
  Add/1 -> Simulink-PS Converter/1, Scope/3, To Workspace/1
  Fcn/1 -> Add/1
  connections:
  Hard_Stop_Knee_L1/LConn1 -- PS-Simulink Converter1/LConn1 -- w/RConn1
  Hard_Stop_Knee_L1/RConn1 -- PS-Simulink Converter3/LConn1 -- PS Add/LConn2
  q/RConn1 -- PS-Simulink Converter2/LConn1
  Simulink-PS Converter1/RConn1 -- PS Add1/LConn2
  PS Add/RConn1 -- PS Add1/LConn1
  PS Add1/RConn1 -- t/RConn1
  Simulink-PS Converter/RConn1 -- PS Add/LConn1
